simulink library "my_filter_lib"  (R2016a)
settings: Solver=ode45  StartTime=0.0  StopTime=10.0  RelTol=1e-3
settings Model: Creator=ebenera  LastModifiedBy=ebenera
settings DataIOCC: LimitDataPoints=on
settings DebuggingCC: AllowSymbolicDim=off

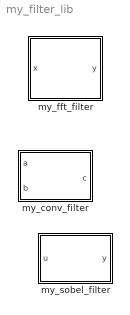
== system my_filter_lib ==
  my_conv_filter : MATLAB Function  TreatAsAtomicUnit=on
  my_fft_filter : Subsystem  TreatAsAtomicUnit=on  mask{shape=valid}
      mask TypeOptions shape: Open the Type Options Editor and enter: | full | same | valid
      mask Display:
      | disp('my_fft');
      | port_label('output', 1, 'ft');
      | port_label('input', 1, 'data');
  my_sobel_filter : MATLAB Function  TreatAsAtomicUnit=on

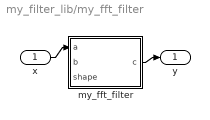
== system my_filter_lib/my_fft_filter ==
  x : Inport
  my_fft_filter : MATLAB Function  TreatAsAtomicUnit=on
  y : Outport
  wires:
  x/1 -> my_fft_filter/1(a)
  my_fft_filter/1(c) -> y/1

== matlab function my_filter_lib/my_conv_filter ==
  data: a input; c output; b input
function c = my_conv(a, b)

c = conv(a, b);

== matlab function my_filter_lib/my_fft_filter/my_fft_filter ==
  data: a input; c output; b input; shape input
function c = my_fft(a, b, shape)
if shape == 1
    c = conv(a, b, 'full');
elseif shape == 2
    c = conv(a, b, 'same');
else
    c = conv(a, b, 'valid');
end

== matlab function my_filter_lib/my_sobel_filter ==
  data: u input; y output
function y = my_sobel(u)

%% "my_sobel_filter" is a MATLAB function
%%  on the  MATLAB path.
y = my_sobel_filter(u);
